simulink model "Modulation_AM_AWGN_SNR"  (R2023a)
settings: Solver=VariableStepAuto  StartTime=0.0  StopTime=1  RelTol=1e-3
libraries: commchan3 x1, dspfdesign x1
settings Model: Creator=Pedro  LastModifiedBy=Pedro

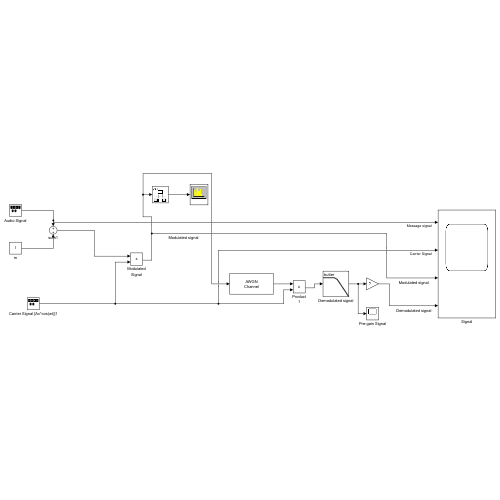
[thumbnail: Simulink's stored preview of the top-level diagram]
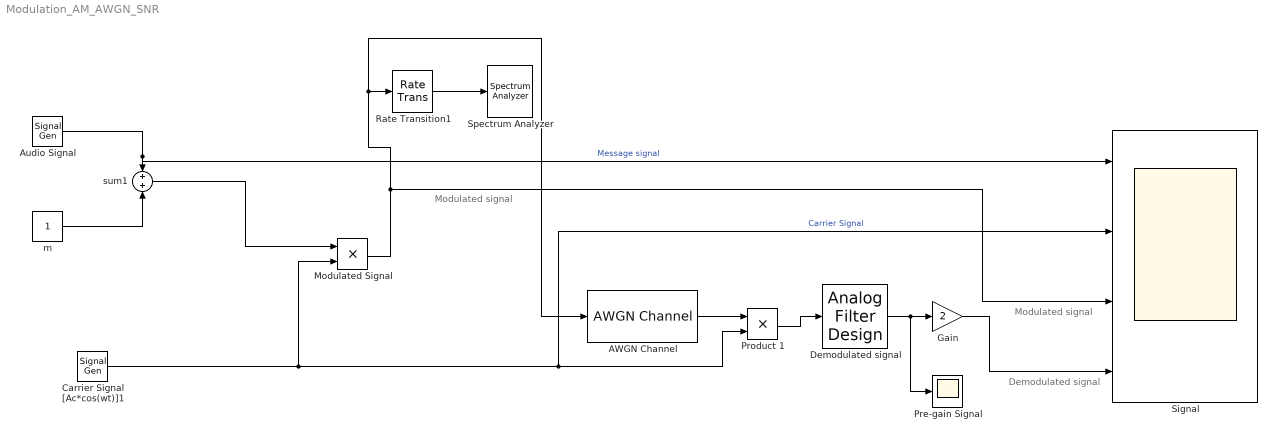
== system Modulation_AM_AWGN_SNR ==
  note: Modulated signal
  note: Demodulated signal
  note: Modulated signal
  AWGN Channel : commchan3/AWGN Channel  LegacyMode=off  NoiseMethod="Signal to noise ratio  (SNR)"  noiseMode="Signal to noise ratio  (SNR)"  EbNo=10  EsNo=10  SNR=20  BitsPerSymbol=1  SignalPower=1  SamplesPerSymbol=1  SymbolPeriod=1  VarianceSource=Parameter  Variance=1  RandomStream=Global stream  Seed=67  SimulateUsing=Code generation
  Audio Signal : SignalGenerator  Frequency=20
  Carrier Signal [Ac*cos(wt)]1 : SignalGenerator  Frequency=110
  Demodulated signal : dspfdesign/Analog Filter Design  method=Butterworth  filttype=Lowpass  N=3  Wlo=43*pi  Whi=80  Rp=2  Rs=40
  Gain : Gain  Gain=2
  Modulated Signal : Product
  Pre-gain Signal : Scope
  Product 1 : Product
  Rate Transition1 : RateTransition  OutPortSampleTime=0.0001
  Signal : Scope  NumInputPorts=4
  Spectrum Analyzer : SpectrumAnalyzer  WindowPosition=[1.000000,41.000000,1280.000000,657.000000,]  ScopeFrameLocation=window  Method=Welch  PlotAsTwoSidedSpectrum=off  Span=5000  CenterFrequency=2500  StartFrequency=0  SpectrumUnits=Watts  YLimits=[-0.05906145,0.53155305]  ColorLimits=[-80 20]  SelectedToolstripTab=spectrumAnalyzerToolstrip.estimationTab
  m : Constant
  sum1 : Sum
  wires:
  m/1 -> sum1/2
  Audio Signal/1 -> sum1/1, Signal/1  "Message signal"
  sum1/1 -> Modulated Signal/1
  Modulated Signal/1 -> Signal/3, Rate Transition1/1, AWGN Channel/1
  Carrier Signal [Ac*cos(wt)]1/1 -> Product 1/2, Signal/2, Modulated Signal/2  "Carrier Signal"
  Rate Transition1/1 -> Spectrum Analyzer/1
  AWGN Channel/1 -> Product 1/1
  Product 1/1 -> Demodulated signal/1
  Demodulated signal/1 -> Pre-gain Signal/1, Gain/1
  Gain/1 -> Signal/4
